simulink model "sim2020_7_21"  (R2017a)
settings: Solver=ode45  StartTime=0.0  StopTime=30  FixedStep=0.05  MaxStep=0.05  RelTol=1e-3
libraries: simulink x2
settings Model: Creator=asus  LastModifiedBy=Lenovo

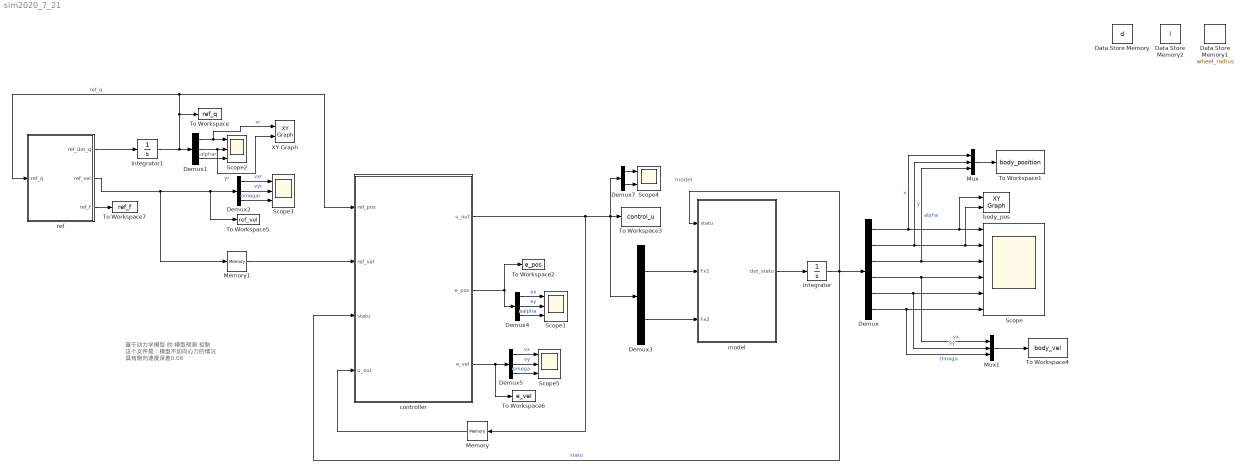
== system sim2020_7_21 ==
  note: 基于动力学模型 的 模型预测 控制
      | 这个文件是：模型不加向心力的情况
      | 具有侧向速度误差0.08
  note: model
  Data Store Memory : DataStoreMemory  DataStoreName=d  ReadBeforeWriteMsg=warning  WriteAfterWriteMsg=warning  WriteAfterReadMsg=warning  ShowAdditionalParam=off  OutDataTypeStr=double
  Data Store Memory1 : DataStoreMemory  DataStoreName=wheel_radius  ReadBeforeWriteMsg=warning  WriteAfterWriteMsg=warning  WriteAfterReadMsg=warning  ShowAdditionalParam=off  OutDataTypeStr=double
  Data Store Memory2 : DataStoreMemory  DataStoreName=l  ReadBeforeWriteMsg=warning  WriteAfterWriteMsg=warning  WriteAfterReadMsg=warning  ShowAdditionalParam=off  OutDataTypeStr=double
  Demux : Demux  Outputs=6
  Demux{1..2,4..5} (4 alike) : Demux  Outputs=3
  Demux3 : Demux  Outputs=2
  Demux7 : Demux  Outputs=2
  Integrator : Integrator  InitialCondition=[2; -2; pi/2; 0.0001; 0; 0]  IgnoreLimit=on
  Integrator1 : Integrator  InitialCondition=[0;0;pi/4]
  Memory : Memory  X0=[0; 0]
  Memory1 : Memory  X0=[2; 0; 0.5]
  Mux : Mux  Inputs=3
  Mux1 : Mux  Inputs=3
  Scope : Scope  NumInputPorts=6
  Scope{1..3,5} (4 alike) : Scope  NumInputPorts=3
  Scope4 : Scope  NumInputPorts=2
  To Workspace : ToWorkspace  VariableName=ref_q  SampleTime=-1
  To Workspace1 : ToWorkspace  VariableName=body_position  SampleTime=-1
  To Workspace2 : ToWorkspace  VariableName=e_pos  SampleTime=-1
  To Workspace3 : ToWorkspace  VariableName=control_u  SampleTime=-1
  To Workspace4 : ToWorkspace  VariableName=body_vel  SampleTime=-1
  To Workspace5 : ToWorkspace  VariableName=ref_vel  SampleTime=-1
  To Workspace6 : ToWorkspace  VariableName=e_vel  SampleTime=-1
  To Workspace7 : ToWorkspace  VariableName=ref_f  SampleTime=-1
  XY Graph : simulink/Sinks/XY Graph  xmin=-10  xmax=10  ymin=-10  ymax=10  st=-1
  body_pos : simulink/Sinks/XY Graph  xmin=-10  xmax=10  ymin=-10  ymax=10  st=-1
  controller : MATLAB Function  TreatAsAtomicUnit=on
  model : MATLAB Function  TreatAsAtomicUnit=on
  ref : MATLAB Function  TreatAsAtomicUnit=on
  wires:
  Demux2/2 -> Scope3/2  "vyr"
  Demux2/1 -> Scope3/1  "vxr"
  Demux4/2 -> Scope1/2  "ey"
  Demux4/3 -> Scope1/3  "ealpha"
  ref/2(ref_vel) -> Memory1/1, To Workspace5/1, Demux2/1
  Integrator/1 -> controller/3(statu), model/1(statu), Demux/1  "statu"
  Demux1/3 -> Scope2/3  "alphar"
  Demux1/1 -> XY Graph/1, Scope2/1  "xr"
  Demux4/1 -> Scope1/1  "ex"
  Demux1/2 -> XY Graph/2, Scope2/2  "yr"
  Demux2/3 -> Scope3/3  "omegar"
  Demux/3 -> Mux/3, Scope/3  "alpha"
  Demux/1 -> Mux/1, body_pos/1, Scope/1  "x"
  Demux/2 -> Mux/2, body_pos/2, Scope/2  "y"
  ref/1(ref_dot_q) -> Integrator1/1
  Integrator1/1 -> ref/1(ref_q), controller/1(ref_pos), To Workspace/1, Demux1/1  "ref_q"
  Demux7/2 -> Scope4/2
  Demux7/1 -> Scope4/1
  model/1(dot_statu) -> Integrator/1
  Demux/4 -> Mux1/1, Scope/4  "vx"
  Demux/5 -> Mux1/2, Scope/5  "vy"
  Demux/6 -> Mux1/3, Scope/6  "Omega"
  Demux3/1 -> model/2(Fx1)
  controller/1(u_out) -> Memory/1, Demux7/1, To Workspace3/1, Demux3/1
  Demux3/2 -> model/3(Fx2)
  Mux1/1 -> To Workspace4/1
  Mux/1 -> To Workspace1/1
  controller/2(e_pos) -> To Workspace2/1, Demux4/1
  Demux5/1 -> Scope5/1  "vx"
  Demux5/2 -> Scope5/2  "vy"
  Demux5/3 -> Scope5/3  "omega"
  controller/3(e_vel) -> To Workspace6/1, Demux5/1
  Memory/1 -> controller/4("u_out ")
  Memory1/1 -> controller/2(ref_vel)
  ref/3(ref_f) -> To Workspace7/1

== matlab function sim2020_7_21/controller ==
  data: ref_pos input; ref_vel input; u_out output; statu input; e_pos output; e_vel output; u_out input
function [u_out, e_pos, e_vel] = my_MPC_controller(ref_pos, ref_vel, statu, u_out)
% 最近修改时间：7.25 
% 基于动力学模型的MPC控制器
% u_out=[fl ; fr]
% ref_vel=[xr yr alphar vr omegar]
% e = [ex ey ealpha]

Nc=15; Np=30; %预测时域Np	控制时域Nc
T=0.05; 

% 测试是否能得到
%    statu=[2; -2; pi/2; 0.001; 0.001; 0.001];
%    u_out=[0; 0];
%    ref_pos=[0;0;pi/4]; ref_vel=[2; 0; 0];  
%% 底盘参数
d = 0.18;	l = 0.16;	m = 24;	Iz = 11.89;	c = 513.6; %轮胎侧偏刚度

%% 状态量                                                                           
x = statu(1);   y = statu(2);  alpha = statu(3); 
vx = statu(4);  vy = statu(5);    omega = statu(6);
                                      
                                                                            
xr=ref_pos(1);  yr=ref_pos(2);  alphar=ref_pos(3);
vxr=ref_vel(1); vyr=ref_vel(2); omegar=ref_vel(3);
                                                                                      
%控制量个数Nu
Nu=size(u_out,1);

%状态量个数Nx
statu_error=[x-xr;   y-yr;   alpha-alphar;  vx-vxr; vy-vyr; omega-omegar]; 

Nx=size(statu_error,1);

% 控制矩阵求解(将连续矩阵转换为离散矩阵，采用近似算法  A=I+T*A(t),B=T*B(t))
% 此处：delta_X=AX+BU ————X=[a-r]=[X_I-Xr;Y_I-Yr;ALPHA_I-ALPHAr]statu_e=A*statu_e+B*u_e   %离散后的模型
    % OUT=delta_X=a-r
A=[ 1, 0, (-vxr*sin(alphar)-vyr*cos(alphar))*T, T*cos(alphar), -T*sin(alphar), 0;
    0, 1, (vxr*cos(alphar)-vyr*sin(alphar))*T,  T*sin(alphar), T*cos(alphar), 0;
    0, 0, 1, 0, 0, T;
    0, 0, 0, 1, 0, 0;
    0, 0, 0, T*(2*c*(vyr+l*omegar))/(m*vxr^2), (-2*c*T)/(m*vxr)+1, (-2*c*l*T)/(m*vxr);
    0, 0, 0, -T*(2*c*l*(vyr+l*omegar))/(Iz*vxr^2), 2*c*l*T/(Iz*vxr), (2*c*l*l*T)/(vxr*Iz)+1;] ; %+0.0001是为了避免分母为零
B=[0 0;
   0 0;
   0 0;
   T/m T/m;
   0 0;
   -T*d/Iz T*d/Iz;];

C = eye(Nx);
% C = [0 0 0 1 0 0;
%      0 0 0 0 1 0;
%      0 0 0 0 0 1];

Error = C * statu_error; % 误差

e_pos=Error(1:Nx/2); %位置误差
e_vel=Error(Nx/2:Nx); %速度误差

% 得到新的X=A_new*X+B_new*delta_u   X=[X;u-ur]
A_new = [A B;zeros(Nu,Nx) eye(Nu)];
B_new = [B;eye(Nu)];
C_new = [C,zeros(Nx,Nu)];
%% 
ur=[0; 0];

statu_new = [Error;u_out-ur];

PHI=zeros(Np*size(C_new*A_new,1),size(A_new,2));
for i=1:1:Np
    PHI( Nx*i-(Nx-1):Nx*i ,:)=C_new*A_new^i;
end

THETA=zeros( Np*size(C_new*B_new,1),  Nc*size(C_new*A_new*B_new ,2) );
for i=1:1:Np
    for j=1:1:Nc
        if j<= i
            THETA( Nx*i-5:Nx*i,Nu*j-1:Nu*j )= C_new*A_new^(i-j)*B_new;
        else
            THETA( Nx*i-5:Nx*i,Nu*j-1:Nu*j ) = zeros( Nx,Nu );
        end
    end
end

% q = [1000 0 0 0 0 0;
%      0 1000 0 0 0 0;
%      0 0 1000 0 0 0;
%      0 0 0 100 0 0;
%      0 0 0 0 500 0;
%      0 0 0 0 0 500;];
%  q = [10 0 0 0 0 0;
%      0 10 0 0 0 0;
%      0 0 10 0 0 0;
%      0 0 0 10 0 0;
%      0 0 0 0 1000 0;
%      0 0 0 0 0 10;];
 q = [10 0 0;
      0 10 0;
      0 0 10;];

Q=zeros(Nx*Np,Nx*Np);
for i=1:Np
    for j=1:Np
        if i==j
            Q(Nx*(i-1)+1:Nx*i , Nx*(i-1)+1:Nx*i) = q;
        end
    end
end

R = 1*eye( Nc*Nu,Nc*Nu);

%% 二次型
p=2;

H = [2*THETA'*Q*THETA+R zeros(Nc*Nu,1);zeros(1,Nc*Nu) p];  %不是对称的 % 前面加了个2

ERROR =PHI*statu_new;  
G = [2*ERROR'*Q*THETA zeros(1)];
P_T = ERROR'*Q*ERROR;

%% 约束条件
%控制量约束
M=tril(ones(Nc));
Im= eye(Nu);
A=kron(M,Im); % U=A*DELTA_U+Ut  中的A

Ut=kron(ones(Nc,1),u_out); %Ut

umin=[-400;-400];  %维数与控制变量的个数相同
umax=[ 400; 400];
Umin=kron(ones(Nc,1),umin);
Umax=kron(ones(Nc,1),umax);
a = [A zeros(Nu*Nc,1);-A zeros(Nu*Nc,1)];
b = [Umax-Ut;-Umin+Ut];

 % 状态增量约束
delta_u_range=10;
delta_Umin = kron((-delta_u_range)*ones(Nu,1),ones(Nc,1)); %速度增量约束
delta_Umax = kron( (delta_u_range)*ones(Nu,1),ones(Nc,1));

lb=[delta_Umin;-2];%（求解方程）状态量下界，包含控制时域内控制增量和松弛因子
ub=[delta_Umax;2];%（求解方程）状态量上界，包含控制时域内控制增量和松弛因子
  
%%
coder.extrinsic('quadprog');
coder.extrinsic('tic');
coder.extrinsic('toc');
tic 
[DELTA_U,fval]=quadprog(H,G,a,b,[],[],lb,ub);
toc

delta_u = zeros(Nu*Nc+1,1);	% 定义类型，存储DELTA_U的mxarray类型数据
delta_u = DELTA_U;
delta_uout = delta_u(1:2)
u_out = delta_uout+u_out

== matlab function sim2020_7_21/model ==
  data: statu input; dot_statu output; wheel_radius data_store_memory; l data_store_memory; d data_store_memory; Fx1 input; Fx2 input
function dot_statu = model(statu, Fx1 , Fx2 )
global wheel_radius d l ;
wheel_radius = 0.330/2;
d = 0.18;
l = 0.16;
m = 24;
Iz = 11.89;
c = 513.6; %轮胎侧偏刚度


x = statu(1);   y = statu(2);   alpha = statu(3);
vx = statu(4);  vy = statu(5);  omega = statu(6);

dot_x = vx*cos(alpha)-vy*sin(alpha);
dot_y = vx*sin(alpha)+vy*cos(alpha);
dot_alpha = omega;
dot_vx = (Fx1+Fx2)/m ;  
dot_vy = (-2*c*(vy+l*omega))/(m*vx) ;
dot_omega = (Fx2-Fx1)*d/(Iz)+(2*c*l*(vy+l*omega))/(Iz*vx);


% Fy1 = -c*(vy-l*omega)/(vx-d*omega);
% Fy2 = -c*(vy-l*omega)/(vx+d*omega);
% 
% dot_x = vx*cos(alpha)-vy*sin(alpha);
% dot_y = vx*sin(alpha)+vy*cos(alpha);
% dot_alpha = omega;
% dot_vx = (Fx1+Fx2)/m + omega*vy;  % add 向心力
% dot_vy = (Fy1+Fy2)/m - omega*vx;
% dot_omega = (Fx2-Fx1)*d/(Iz)-(Fy1+Fy2)*l/(Iz);


% 状态【x y alpha vx vy omega】
dot_statu = [dot_x; dot_y; dot_alpha; dot_vx; dot_vy; dot_omega]; 

end

== matlab function sim2020_7_21/ref ==
  data: ref_q input; ref_dot_q output; ref_vel output; ref_f output
function [ref_dot_q,ref_vel,ref_f] = fcn(ref_q)
xr=ref_q(1);
yr=ref_q(2);
alphar=ref_q(3);

vxr=1;
vyr=0;
omegar=0.5;

ref_vel=[vxr;vyr;omegar];

dotx = vxr*cos(alphar) - vyr*sin(alphar);
doty = vxr*sin(alphar) + vyr*sin(alphar);
dotalpha = omegar;
ref_dot_q=[dotx;doty;dotalpha];

ref_f=[0;0];
end
